simulink model "algLoopMultipleSolutions"  (R2018a)
settings: Solver=ode45  StartTime=0.0  StopTime=10.0  RelTol=1e-12  EnableMultiTasking=on
settings Model: Creator=jrivitus  LastModifiedBy=bneiswan
settings SolverCC: ShapePreserveControl=EnableAll  AlgebraicLoopSolver=LineSearch
settings DataIOCC: LimitDataPoints=on  SaveFormat=Array
settings OptimizationCC: ExpressionDepthLimit=2147483647  LifeSpan=inf
settings DebuggingCC: UnderspecifiedInitializationDetection=Classic  MergeDetectMultiDrivingBlocksExec=none  ParameterPrecisionLossMsg=none  FcnCallInpInsideContextMsg=warning  AllowSymbolicDim=off  StateNameClashWarn=warning  SFUnexpectedBacktrackingDiag=warning  SFNoUnconditionalDefaultTransitionDiag=warning  SFExecutionAtInitializationDiag=none
settings HardwareCC: ProdBitPerPointer=32  ProdBitPerSizeT=32  ProdBitPerPtrDiffT=32  ProdLargestAtomicFloat=None  ProdIntDivRoundTo=Undefined  ProdEndianess=Unspecified  ProdWordSize=32  ProdHWDeviceType=32-bit Generic
settings ModelReferenceCC: PropagateSignalLabelsOutOfModel=off
settings CodeAppCC: StateflowObjectComments=on
settings GRTTargetCC: TargetLangStandard=C89/C90 (ANSI)  GeneratePreprocessorConditionals=Disable all  CombineOutputUpdateFcns=off  GRTInterface=on
settings ConfigComp: CovMetricSettings=dw  CovHtmlReporting=on  CovSaveCumulativeToWorkspaceVar=on  CovSaveSingleToWorkspaceVar=on  CovExternalEMLEnable=off  CovSFcnEnable=off

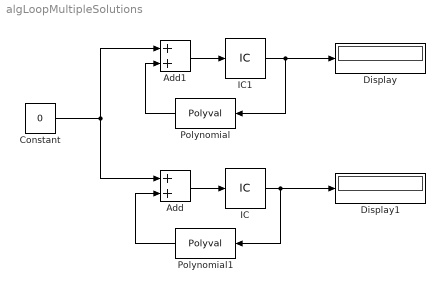
== system algLoopMultipleSolutions ==
  Add : Sum
  Add1 : Sum
  Constant : Constant  Value=0
  Display : Display
  Display1 : Display
  IC : InitialCondition  Value=-100
  IC1 : InitialCondition  Value=100
  Polynomial : Polyval  Coefs=[-1 -5 1]
      settings: AttributesFormatString="Coefficients:  %<Coefs>"
  Polynomial1 : Polyval  Coefs=[-1 -5 1]
      settings: AttributesFormatString="Coefficients:  %<Coefs>"
  wires:
  Polynomial1/1 -> Add/2
  Add/1 -> IC/1
  IC/1 -> Polynomial1/1, Display1/1
  Polynomial/1 -> Add1/2
  Add1/1 -> IC1/1
  IC1/1 -> Polynomial/1, Display/1
  Constant/1 -> Add1/1, Add/1
